simulink model "BEML_EMU"  (R2019b)
settings: configuration reference "ConfigSet_SimIntegration" (kept outside this file)
model workspace (MAT data in the model file):
  BrakesSampleTime = 0.01
  ConfigSampleTime = 0.05
  CouplingSampleTime = 0.05
  DoorsSampleTime = 0.05
  DynamicsSampleTime = 0.001
  ElectricalSampleTime = 0.05
  PRM_SimIntegration : Simulink.Parameter (value not decoded)
  PantographSampleTime = 0.05
  PneumaticsSampleTime = 0.01
  SampleTime = 0.001
  TractionSampleTime = 0.01
undefined symbols (not defined in the file): Acceleration, AngularAcceleration, AngularVelocity, BrakeFadeEnable, Brakes, BrakeShoeCoefficientCalculationMethod, BrakeShoeFrictionCoeff, BrakeTemperatureEnable, Common, DampingAdjustmentDesignMass, DavisCoeffA1, DavisCoeffA2, DavisCoeffB1, DavisCoeffB2, DavisCoefficients, DavisCoeffLeadCarC, DavisCoeffTailCarC, DiscIntNeverNeededParam, Doors, DragCalculationMethod, Dynamics, Effects, Electrical, EnableDampingAdjustmentByMass, Environment, Equipment, ExternalEffects, H, HasMotor, HasPanto, HornActivation, IsFirstVehicle, IsLastVehicle, isLeft, IsNonCab, LateralJolt, Location, LongitudinalJolt, MaxVehicles, MotionBaseSafetyCutout, OrientationDCM, P, Pantograph, Pneumatics, PneumaticsPoweredPanto, R, Traction, Transform, Tuning, UnitConfig, Velocity, VerticalJolt, VerticalJoltDown, VigilanceIntervention
libraries: simulink x35, IOStateMachinesLib x26, TestBenchLib x6, LatchesLib x3, BEML_EMU_BrakesInput_Lib x1, BEML_EMU_CBTCInterface_Lib x1, BEML_EMU_Couplers_Lib x1, BEML_EMU_DoorsInput_Lib x1, BEML_EMU_DynamicsInput_Lib x1, BEML_EMU_ElectricalInput_Lib x1, BEML_EMU_PantographInput_Lib x1, BEML_EMU_PneumaticsInput_Lib x1
(part 2 of 6)

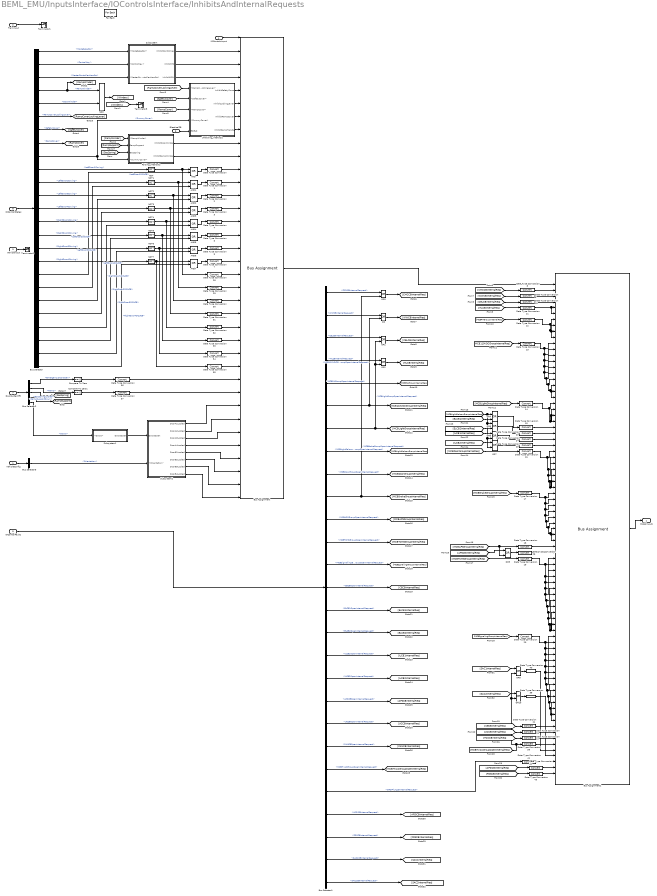
== system BEML_EMU/InputsInterface/IOControlsInterface/InhibitsAndInternalRequests ==
  VehicleConfig : Inport  Partition=on  PartitionDimension=1  PartitionWidth=1  PartitionOffset=0
  TrainInput : Inport  Port=2
  VehicleInput : Inport  Port=3  Partition=on  PartitionDimension=1  PartitionWidth=1  PartitionOffset=0
  IOControlsInput : Inport  Port=4  Partition=on  PartitionDimension=1  PartitionWidth=1  PartitionOffset=0
  IOControlFaults : Inport  Port=5  Partition=on  PartitionDimension=1  PartitionWidth=1  PartitionOffset=0
  ElectricalFB : Inport  Port=6  Partition=on  PartitionDimension=1  PartitionWidth=1  PartitionOffset=0
  DoorSystemFB : Inport  Port=7  Partition=on  PartitionDimension=1  PartitionWidth=1  PartitionOffset=0
  IOControlStates : Inport  Port=8  Partition=on  PartitionDimension=1  PartitionWidth=1  PartitionOffset=0
  AND{,1..7} (8 alike) : Logic  Operator=OR  AllPortsSameDT=off  OutDataTypeStr=boolean
  Bus Assignment : BusAssignment  AssignedSignals=ControlKey.Inhibit,ModeSelector.Inhibit,MasterControllerHandle.Inhibit,SafetyCover.Inhibit,RampCoverLockingLever.Inhibit,RampCover.Inhibit,RampHandle.Inhibit,DoorWinder.Inhibit,RampWinder.Inhibit,LeftDoor1EED.Inhibit,LeftDoor2EED.Inhibit,LeftDoor3EED.Inhibit,LeftDoor4EED.Inhibit,RightDoor1EED.Inhibit,RightDoor2EED.Inhibit,RightDoor3EED.Inhibit,RightDoor4EED.Inhibit,LeftDoor1DCUCB.Inhibit,LeftDoor2DCUCB.Inhibit,LeftDoor3DCUCB.Inhibit,LeftDoor4DCUCB.Inhibit,RightDoor1DCUCB.Inhibit,RightDoor2DCUCB.Inhibit,RightDoor3DCUCB.Inhibit,RightDoor4DCUCB.Inhibit,EmergencyDoorGasSpring.Inhibit,RampMiddleSupport.Inhibit,LeftDoor1Lockout.Inhibit,LeftDoor2Lockout.Inhibit,LeftDoor3Lockout.Inhibit,LeftDoor4Lockout.Inhibit,RightDoor1Lockout.Inhibit,RightDoor2Lockout.Inhibit,RightDoor3Lockout.Inhibit,RightDoor4Lockout.Inhibit
  Bus Assignment1 : BusAssignment  AssignedSignals=CMCCB.InternalRequest,WWCB.InternalRequest,CELCB.InternalRequest,HLLCB.InternalRequest,HLRCB.InternalRequest,OCCB1.InternalRequest,OCCB2.InternalRequest,PISCB1.InternalRequest,PISCB2.InternalRequest,TBCCB1.InternalRequest,TBCCB2.InternalRequest,SSICB.InternalRequest,HCB.InternalRequest,POCB.InternalRequest,TVDUCB.InternalRequest,ODDCB.InternalRequest,WIFICB.InternalRequest,WFLCB.InternalRequest,VCBCB.InternalRequest,MLCB.InternalRequest,TLLCB.InternalRequest,TLRCB.InternalRequest,CILCB.InternalRequest,ELCB1.InternalRequest,ELCB2.InternalRequest,ILCB1.InternalRequest,ILCB2.InternalRequest,LDRCB.InternalRequest,LDLCB.InternalRequest,DLCB.InternalRequest,DRCB.InternalRequest,LDICB.InternalRequest,DPLCB.InternalRequest,EDCB.InternalRequest,BLCB.InternalRequest,ZVBACB.InternalRequest,EBLR1CB.InternalRequest,EBLR2CB.InternalRequest,EBMVCB.InternalRequest,PBCB.InternalRequest,BECUCB1.InternalRequest,BECUCB2.InternalRequest,BECUCB3.InternalRequest,BCGCB.InternalRequest,APSCB.InternalRequest,TDICB.InternalRequest,ERCB.InternalRequest,TBNCB.InternalRequest,CSCCB.InternalRequest,CSBCB.InternalRequest,CSACB.InternalRequest,CDUCB.InternalRequest,DIOCB2.InternalRequest,DIOCB1.InternalRequest,SIOCB1.InternalRequest,SIOCB2.InternalRequest,RIO1CB.InternalRequest,RIO2CB.InternalRequest,TRIVCB.InternalRequest,VIO2CB.InternalRequest,VIO1CB.InternalRequest,PPU3CB.InternalRequest,PPU2CB.InternalRequest,PPU1CB.InternalRequest,C1CB.InternalRequest,NBCB.InternalRequest,MMCB.InternalRequest,CRSBCB.InternalRequest,DMICB.InternalRequest,TWVCB.InternalRequest,CBTCCB1.InternalRequest,NVICB.InternalRequest,CCNVIO1CB.InternalRequest,CECB.InternalRequest,VCCBOrUCCB.InternalRequest,PANCB.InternalRequest,CBFCCB.InternalRequest,SAC1CCB.InternalRequest,SAC2CCB.InternalRequest,ORDPlunger.InternalRequest,APSICB.InternalRequest,FDSCB.InternalRequest
  Bus Selector : BusSelector  OutputSignals=ModeSelector,ControlKey,MasterControllerHandle,RampWinder,DoorWinder,RampCoverLockingLever,SafetyCover,RampCover,DummyCover,LeftDoor1Coving,LeftDoor2Coving,LeftDoor3Coving,LeftDoor4Coving,RightDoor1Coving,RightDoor2Coving,RightDoor3Coving,RightDoor4Coving,LeftDoor1DCUCB,LeftDoor2DCUCB,LeftDoor3DCUCB,LeftDoor4DCUCB,RightDoor1DCUCB,RightDoor2DCUCB,RightDoor3DCUCB,RightDoor4DCUCB
  Bus Selector1 : BusSelector  OutputSignals=CCMCBInternalRequest,WWCBInternalRequest,CELCBInternalRequest,HLCBInternalRequest,MCBPAGroupOpenInternalRequest,MCB110VDCGroupOpenInternalRequest,MCBLightGroupOpenInternalRequest,MCBLightSaloonGroupOpenInternalRequest,MCBDoorGroupOpenInternalRequest,MCBBrakeGroupOpenInternalRequest,MCBAPSGroupOpenInternalRequest,MCBTCMSGroupOpenInternalRequest,MCBSignallingGroupOpenInternalRequest,CECBOpenInternalRequest,ELCB1OpenInternalRequest,ELCB2OpenInternalRequest,ILCB1OpenInternalRequest,ILCB2OpenInternalRequest,APSCBOpenInternalRequest,UCCBOpenInternalRequest,PANCBOpenInternalRequest,MCBHVACGroupOpenInternalRequest,ORDPlungerInternalRequest,APSICBInternalRequest,FDSCBInternalRequest,SAC1CBInternalRequest,SAC2CBInternalRequest
  Bus Selector2 : BusSelector  OutputSignals=EmergencyDoor.EmergencyDoorOpen,EmergencyDoor.Ramp,EmergencyDoor.GasSpringLocked,EmergencyDoor.RampSupportDown,Doors
  Bus Selector3 : BusSelector  OutputSignals=Common.Orientation
  Compare To Zero : simulink/Logic and Bit Operations/Compare To Zero  relop===  OutDataTypeStr=boolean
  Compare To Zero1 : simulink/Logic and Bit Operations/Compare To Zero  relop===  OutDataTypeStr=boolean
  Data Type Conversion{,1..43} (44 alike) : DataTypeConversion
  Folding_Interlocks : Subsystem
  For Each : ForEach  DisableCoverage=on
  NOR : Logic  Operator=NOR  AllPortsSameDT=off  OutDataTypeStr=boolean
  NOT{,1..7} (8 alike) : Logic  Operator=NOT  AllPortsSameDT=off  OutDataTypeStr=boolean
  OR{,1..10} (11 alike) : Logic  Operator=OR  AllPortsSameDT=off  OutDataTypeStr=boolean
  Subsystem : Subsystem
  Subsystem1 : Subsystem
  Subsystem2 : Subsystem
  Terminator1 : Terminator
  Terminator2 : Terminator
  Terminator3 : Terminator
  Unfolding_interlocks : Subsystem
  ModelInputs : Outport  ConcatenationDimension=1
  wires:
  AND4/1 -> Data Type Conversion4/1
  AND/1 -> Data Type Conversion/1
  IOControlStates/1 -> Bus Selector/1
  Bus Selector/17 -> NOT7/1  "<RightDoor4Coving>"
  Bus Selector/11 -> NOT1/1  "<LeftDoor2Coving>"
  AND5/1 -> Data Type Conversion5/1
  AND1/1 -> Data Type Conversion1/1
  AND6/1 -> Data Type Conversion6/1
  AND2/1 -> Data Type Conversion2/1
  AND3/1 -> Data Type Conversion3/1
  Bus Selector/10 -> NOT/1  "<LeftDoor1Coving>"
  Bus Selector/4 -> [RampWinder], NOR/1  "<RampWinder>"
  Bus Selector/13 -> NOT3/1  "<LeftDoor4Coving>"
  Bus Selector/12 -> NOT2/1  "<LeftDoor3Coving>"
  Bus Selector/14 -> NOT4/1  "<RightDoor1Coving>"
  Bus Selector/16 -> NOT6/1  "<RightDoor3Coving>"
  Bus Selector/15 -> NOT5/1  "<RightDoor2Coving>"
  AND7/1 -> Data Type Conversion7/1
  Folding_Interlocks/2(InhibitRampWinder) -> Bus Assignment/10
  Folding_Interlocks/1(InhibitDoorWinder) -> Bus Assignment/9
  Bus Assignment/1 -> Bus Assignment1/1
  IOControlFaults/1 -> Bus Selector1/1
  Subsystem/2(InhibitMS) -> Bus Assignment/3
  TrainInput/1 -> Terminator1/1
  Unfolding_interlocks/3(InhibitRampCover) -> Bus Assignment/7
  Bus Selector/2 -> Subsystem/2(<ControlKey>)  "<ControlKey>"
  Subsystem/1(InhibitControlKey) -> Bus Assignment/2
  VehicleInput/1 -> Terminator2/1
  VehicleConfig/1 -> Bus Selector3/1
  Bus Selector/5 -> NOR/2  "<DoorWinder>"
  Subsystem/3(InhibitMCH) -> Bus Assignment/4
  IOControlsInput/1 -> Bus Assignment/1
  Bus Selector/3 -> Subsystem/3(<MasterControllerHandle>)  "<MasterControllerHandle>"
  Unfolding_interlocks/1(InhibitSafetyCover) -> Bus Assignment/5
  Unfolding_interlocks/4(InhibitRampHandle) -> Bus Assignment/8
  Unfolding_interlocks/2(InhibitLockingLever) -> Bus Assignment/6
  Bus Selector/9 -> Unfolding_interlocks/4(<DummyCover>), Folding_Interlocks/4(<DummyCover>)  "<DummyCover>"
  Bus Selector/1 -> Subsystem/1(<ModeSelector>)  "<ModeSelector>"
  NOR/1 -> [Winders]
  [Winders] -> Terminator3/1
  [RampWinder] -> Folding_Interlocks/1(<RampWinder>)
  Bus Selector/6 -> [RampCoverLockingLever]  "<RampCoverLockingLever>"
  [RampCoverLockingLever] -> Unfolding_interlocks/1(<RampCoverLockingLever>)
  Bus Selector/7 -> [SafetyCover]  "<SafetyCover>"
  Bus Selector/8 -> [RampCover]  "<RampCover>"
  [SafetyCover] -> Unfolding_interlocks/2(<SafetyCover>)
  [RampCover] -> Unfolding_interlocks/3(<RampCover>)
  Data Type Conversion/1 -> Bus Assignment/11
  Data Type Conversion1/1 -> Bus Assignment/12
  Data Type Conversion2/1 -> Bus Assignment/13
  Data Type Conversion3/1 -> Bus Assignment/14
  Data Type Conversion4/1 -> Bus Assignment/15
  Data Type Conversion5/1 -> Bus Assignment/16
  Data Type Conversion6/1 -> Bus Assignment/17
  Data Type Conversion7/1 -> Bus Assignment/18
  Bus Selector1/1 -> OR3/1  "<CCMCBInternalRequest>"
  Data Type Conversion8/1 -> Bus Assignment1/2
  ElectricalFB/1 -> Unfolding_interlocks/5(EDELR)
  Bus Selector1/2 -> OR/1  "<WWCBInternalRequest>"
  Bus Selector1/3 -> OR1/1  "<CELCBInternalRequest>"
  Data Type Conversion9/1 -> Bus Assignment1/3
  Data Type Conversion10/1 -> Bus Assignment1/4
  Bus Selector1/4 -> OR2/1  "<HLCBInternalRequest>"
  Data Type Conversion11/1 -> Bus Assignment1/6, Bus Assignment1/5
  Bus Selector1/5 -> [MCBPAGroupInternalReq]  "<MCBPAGroupOpenInternalRequest>"
  Bus Assignment1/1 -> ModelInputs/1
  Bus Selector1/6 -> OR/2, [MCB110VDCGroupInternalReq]  "<MCB110VDCGroupOpenInternalRequest>"
  Bus Selector1/7 -> OR1/2, OR2/2, [MCBLightGroupInternalReq]  "<MCBLightGroupOpenInternalRequest>"
  Bus Selector1/8 -> [MCBLightSaloonGroupInternalReq]  "<MCBLightSaloonGroupOpenInternalRequest>"
  Bus Selector1/9 -> [MCBDoorGroupInternalReq]  "<MCBDoorGroupOpenInternalRequest>"
  Bus Selector1/10 -> OR3/2, [MCBBrakeGroupInternalReq]  "<MCBBrakeGroupOpenInternalRequest>"
  Bus Selector1/11 -> [MCBAPSGroupInternalReq]  "<MCBAPSGroupOpenInternalRequest>"
  Bus Selector1/12 -> [MCBTCMSGroupInternalReq]  "<MCBTCMSGroupOpenInternalRequest>"
  Bus Selector1/13 -> [MCBSgnalingGroupInternalReq]  "<MCBSignallingGroupOpenInternalRequest>"
  OR/1 -> [WWCBInternalReq]
  OR1/1 -> [CELCBInternalReq]
  OR2/1 -> [HLCBInternalReq]
  OR3/1 -> [CMCCBInternalReq]
  [CMCCBInternalReq] -> Data Type Conversion8/1
  [WWCBInternalReq] -> Data Type Conversion9/1
  [HLCBInternalReq] -> Data Type Conversion11/1
  [CELCBInternalReq] -> Data Type Conversion10/1
  [MCBPAGroupInternalReq] -> Data Type Conversion12/1
  Data Type Conversion12/1 -> Bus Assignment1/9, Bus Assignment1/10, Bus Assignment1/8, Bus Assignment1/7
  [MCB110VDCGroupInternalReq] -> Data Type Conversion13/1
  Data Type Conversion13/1 -> Bus Assignment1/18, Bus Assignment1/19, Bus Assignment1/20, Bus Assignment1/17, Bus Assignment1/16, Bus Assignment1/15, Bus Assignment1/14, Bus Assignment1/13, Bus Assignment1/12, Bus Assignment1/11
  [MCBLightGroupInternalReq] -> Data Type Conversion14/1
  Data Type Conversion14/1 -> Bus Assignment1/22, Bus Assignment1/23, Bus Assignment1/24, Bus Assignment1/21
  OR4/1 -> Data Type Conversion15/1
  [MCBDoorGroupInternalReq] -> Data Type Conversion16/1
  Data Type Conversion16/1 -> Bus Assignment1/30, Bus Assignment1/31, Bus Assignment1/32, Bus Assignment1/33, Bus Assignment1/35, Bus Assignment1/34, Bus Assignment1/29
  [MCBBrakeGroupInternalReq] -> Data Type Conversion17/1
  Data Type Conversion17/1 -> Bus Assignment1/38, Bus Assignment1/40, Bus Assignment1/41, Bus Assignment1/42, Bus Assignment1/43, Bus Assignment1/44, Bus Assignment1/39, Bus Assignment1/37, Bus Assignment1/36
  [MCBAPSGroupInternalReq] -> OR9/2, Data Type Conversion18/1
  Data Type Conversion18/1 -> Bus Assignment1/45
  [MCBTCMSGroupInternalReq] -> Data Type Conversion19/1
  Data Type Conversion19/1 -> Bus Assignment1/48, Bus Assignment1/49, Bus Assignment1/50, Bus Assignment1/51, Bus Assignment1/52, Bus Assignment1/53, Bus Assignment1/54, Bus Assignment1/55, Bus Assignment1/56, Bus Assignment1/57, Bus Assignment1/58, Bus Assignment1/59, Bus Assignment1/47
  Data Type Conversion20/1 -> Bus Assignment1/62, Bus Assignment1/63, Bus Assignment1/64, Bus Assignment1/65, Bus Assignment1/66, Bus Assignment1/67, Bus Assignment1/68, Bus Assignment1/69, Bus Assignment1/70, Bus Assignment1/71, Bus Assignment1/73, Bus Assignment1/72, Bus Assignment1/74, Bus Assignment1/61, Bus Assignment1/60
  [MCBSgnalingGroupInternalReq] -> Data Type Conversion20/1
  Bus Selector1/14 -> [CECBInternalReq]  "<CECBOpenInternalRequest>"
  Bus Selector1/15 -> [ELCB1InternalReq]  "<ELCB1OpenInternalRequest>"
  Bus Selector1/16 -> [ELCB2InternalReq]  "<ELCB2OpenInternalRequest>"
  Bus Selector1/17 -> [ILCB1InternalReq]  "<ILCB1OpenInternalRequest>"
  Bus Selector1/18 -> [ILCB2InternalReq]  "<ILCB2OpenInternalRequest>"
  Bus Selector1/19 -> [APSCBInternalReq]  "<APSCBOpenInternalRequest>"
  Bus Selector1/20 -> [UCCBInternalReq]  "<UCCBOpenInternalRequest>"
  [CECBInternalReq] -> Data Type Conversion21/1
  Data Type Conversion21/1 -> Bus Assignment1/75
  [UCCBInternalReq] -> Data Type Conversion22/1
  Data Type Conversion22/1 -> Bus Assignment1/76
  Data Type Conversion15/1 -> Bus Assignment1/25
  Data Type Conversion23/1 -> Bus Assignment1/26
  Data Type Conversion24/1 -> Bus Assignment1/27
  Data Type Conversion25/1 -> Bus Assignment1/28
  OR5/1 -> Data Type Conversion23/1
  OR6/1 -> Data Type Conversion24/1
  OR7/1 -> Data Type Conversion25/1
  [MCBLightSaloonGroupInternalReq] -> OR7/2, OR6/2, OR5/1, OR4/1
  [ELCB1InternalReq] -> OR4/2
  [ELCB2InternalReq] -> OR5/2
  [ILCB1InternalReq] -> OR6/1
  [ILCB2InternalReq] -> OR7/1
  Data Type Conversion26/1 -> Bus Assignment1/46
  OR9/1 -> Data Type Conversion26/1
  [APSCBInternalReq] -> OR9/1
  Bus Selector1/21 -> [PANCBInternalReq]  "<PANCBOpenInternalRequest>"
  [PANCBInternalReq] -> Data Type Conversion27/1
  Data Type Conversion27/1 -> Bus Assignment1/77
  Bus Selector/18 -> AND/2  "<LeftDoor1DCUCB>"
  Bus Selector/19 -> AND1/2  "<LeftDoor2DCUCB>"
  Bus Selector/20 -> AND2/2  "<LeftDoor3DCUCB>"
  Bus Selector/21 -> AND3/2  "<LeftDoor4DCUCB>"
  Bus Selector/22 -> AND4/2  "<RightDoor1DCUCB>"
  Bus Selector/23 -> AND5/2  "<RightDoor2DCUCB>"
  Bus Selector/24 -> AND6/2  "<RightDoor3DCUCB>"
  Bus Selector/25 -> AND7/2  "<RightDoor4DCUCB>"
  NOT/1 -> Data Type Conversion28/1, AND/1
  NOT1/1 -> Data Type Conversion29/1, AND1/1
  NOT2/1 -> Data Type Conversion30/1, AND2/1
  NOT3/1 -> Data Type Conversion31/1, AND3/1
  NOT4/1 -> Data Type Conversion32/1, AND4/1
  NOT5/1 -> Data Type Conversion33/1, AND5/1
  NOT6/1 -> Data Type Conversion34/1, AND6/1
  NOT7/1 -> Data Type Conversion35/1, AND7/1
  Data Type Conversion28/1 -> Bus Assignment/19
  Data Type Conversion29/1 -> Bus Assignment/20
  Data Type Conversion30/1 -> Bus Assignment/21
  Data Type Conversion31/1 -> Bus Assignment/22
  Data Type Conversion32/1 -> Bus Assignment/23
  Data Type Conversion33/1 -> Bus Assignment/24
  Data Type Conversion34/1 -> Bus Assignment/25
  Data Type Conversion35/1 -> Bus Assignment/26
  [RampSupport] -> Folding_Interlocks/2(RampSupport)
  [GasSpring] -> Folding_Interlocks/3(GasSpring)
  Compare To Zero/1 -> Data Type Conversion36/1
  Compare To Zero1/1 -> Data Type Conversion37/1
  Data Type Conversion36/1 -> Bus Assignment/27
  Data Type Conversion37/1 -> Bus Assignment/28
  Bus Selector1/22 -> [MCBHVACGroupOpenInternalReq]  "<MCBHVACGroupOpenInternalRequest>"
  Data Type Conversion39/1 -> Bus Assignment1/78
  DoorSystemFB/1 -> Bus Selector2/1
  Bus Selector2/1 -> Compare To Zero/1  "<EmergencyDoorOpen>"
  Bus Selector2/2 -> Compare To Zero1/1  "<Ramp>"
  Bus Selector2/3 -> [GasSpring]  "<GasSpringLocked>"
  Bus Selector2/4 -> [RampSupport]  "<RampSupportDown>"
  Bus Selector2/5 -> Subsystem1/1(<Doors>)  "<Doors>"
  Subsystem1/1(DoorsOpen) -> Subsystem2/1(DoorsOpen)
  Bus Selector3/1 -> Subsystem2/2(<Orientation>)  "<Orientation>"
  Subsystem2/1(DoorA1Locked) -> Bus Assignment/29
  Subsystem2/2(DoorA2Locked) -> Bus Assignment/30
  Subsystem2/3(DoorA3Locked) -> Bus Assignment/31
  Subsystem2/4(DoorA4Locked) -> Bus Assignment/32
  Subsystem2/5(DoorB1Locked) -> Bus Assignment/33
  Subsystem2/6(DoorB2Locked) -> Bus Assignment/34
  Subsystem2/7(DoorB3Locked) -> Bus Assignment/35
  Subsystem2/8(DoorB4Locked) -> Bus Assignment/36
  Bus Selector1/23 -> Data Type Conversion41/1  "<ORDPlungerInternalRequest>"
  Data Type Conversion41/1 -> Bus Assignment1/81
  Bus Selector1/24 -> [APSICBInternalReq]  "<APSICBInternalRequest>"
  Bus Selector1/25 -> [FDSCBInternalReq]  "<FDSCBInternalRequest>"
  Bus Selector1/26 -> [SAC1InternalReq]  "<SAC1CBInternalRequest>"
  Bus Selector1/27 -> [SAC2InternalReq]  "<SAC2CBInternalRequest>"
  [APSICBInternalReq] -> Data Type Conversion42/1
  [FDSCBInternalReq] -> Data Type Conversion43/1
  [SAC1InternalReq] -> OR8/1
  [SAC2InternalReq] -> OR10/1
  OR8/1 -> Data Type Conversion40/1
  OR10/1 -> Data Type Conversion38/1
  [MCBHVACGroupOpenInternalReq] -> OR10/2, OR8/2, Data Type Conversion39/1
  Data Type Conversion38/1 -> Bus Assignment1/80
  Data Type Conversion40/1 -> Bus Assignment1/79
  Data Type Conversion42/1 -> Bus Assignment1/82
  Data Type Conversion43/1 -> Bus Assignment1/83

== system BEML_EMU/InputsInterface/VehicleConfigProcessing/VehicleConfigInterface ==
  VehicleConfig : Inport
  TrainInput : Inport  Port=2
  Enable : EnablePort
  Data Type Conversion : DataTypeConversion
  Enumerated Voltages : VectorOperationsLib/Enumerated Voltages
      settings: SourceProductName=Sydac Utilities
  Max : MinMax  Function=max
  Product : Product
  Terminator : Terminator
  Unit Delay : UnitDelay  SampleTime=-1  HasFrameUpgradeWarning=on
  VehicleConfigInterface : Subsystem
  VehicleEnabled : Subsystem
  VehicleConfigProcessed : Outport  SourceOfInitialOutputValue=Input signal  VectorParamsAs1DForOutWhenUnconnected=off
  wires:
  VehicleConfigInterface/1(VehicleConfigProcessed) -> VehicleConfigProcessed/1
  VehicleConfig/1 -> VehicleEnabled/1(VehicleConfig), VehicleConfigInterface/1(VehicleConfig)
  TrainInput/1 -> VehicleConfigInterface/6(TrainInput)
  VehicleEnabled/2(VehicleEnabledDown) -> VehicleConfigInterface/3(VehicleDownEnabled)
  VehicleEnabled/1(VehicleEnabledUp) -> VehicleConfigInterface/2(VehicleUpEnabled)
  VehicleConfigInterface/3(UnitConn) -> Enumerated Voltages/1
  Enumerated Voltages/1 -> Product/2
  Product/1 -> Data Type Conversion/1
  VehicleEnabled/3(VehicleClassDown) -> VehicleConfigInterface/4(ClassDown)
  VehicleEnabled/4(VehicleClassUp) -> VehicleConfigInterface/5(ClassUp)
  Unit Delay/1 -> VehicleConfigInterface/7(UnitID), Max/1
  VehicleConfigInterface/2(Enable) -> Product/1
  Data Type Conversion/1 -> Terminator/1, Unit Delay/1
  Max/1 -> VehicleConfigInterface/8(MaxUnits)

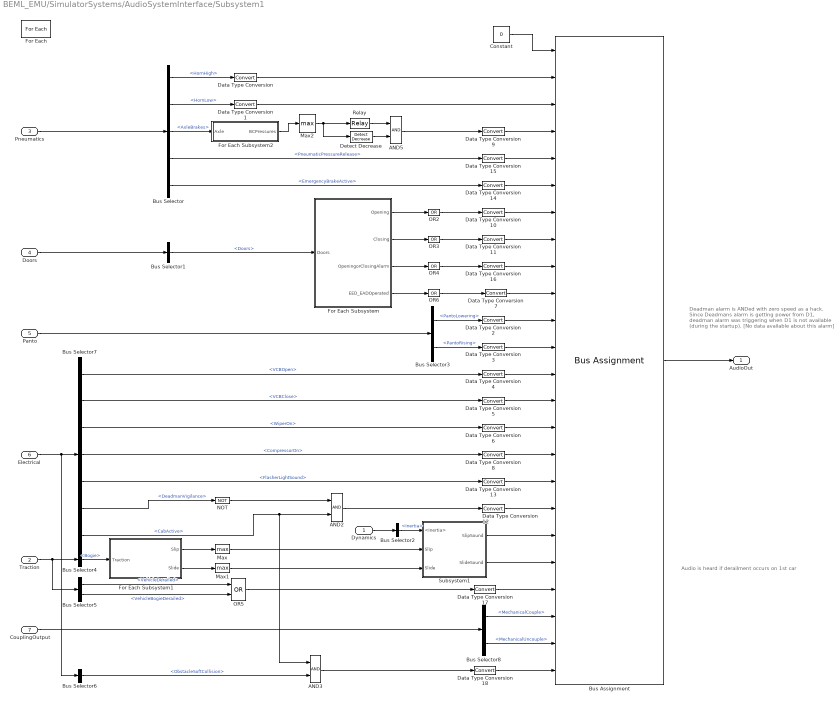
== system BEML_EMU/SimulatorSystems/AudioSystemInterface/Subsystem1 ==
  note: Audio is heard if derailment occurs on 1st car
  note: Deadman alarm is ANDed with zero speed as a hack.
      | Since Deadmans alarm is getting power from D1,
      | deadman alarm was triggering when D1
      | is not available (during the startup).
      | [No data available about this alarm]
  Dynamics : Inport  Partition=on  PartitionDimension=1  PartitionWidth=1  PartitionOffset=0
  Traction : Inport  Port=2  Partition=on  PartitionDimension=1  PartitionWidth=1  PartitionOffset=0
  Pneumatics : Inport  Port=3  Partition=on  PartitionDimension=1  PartitionWidth=1  PartitionOffset=0
  Doors : Inport  Port=4  Partition=on  PartitionDimension=1  PartitionWidth=1  PartitionOffset=0
  Panto : Inport  Port=5  Partition=on  PartitionDimension=1  PartitionWidth=1  PartitionOffset=0
  Electrical : Inport  Port=6  Partition=on  PartitionDimension=1  PartitionWidth=1  PartitionOffset=0
  CouplingOutput : Inport  Port=7  Partition=on  PartitionDimension=1  PartitionWidth=1  PartitionOffset=0
  AND2 : Logic  AllPortsSameDT=off  OutDataTypeStr=boolean
  AND3 : Logic  AllPortsSameDT=off  OutDataTypeStr=boolean
  AND5 : Logic  AllPortsSameDT=off  OutDataTypeStr=boolean
  Bus Assignment : BusAssignment  AssignedSignals=HornHigh,HornLow,AirBrakeRelease,PneumaticPressureRelease,EmergencyBrakeApplicationSound,SaloonDoorOpeningBuzzer,SaloonDoorClosingBuzzer,DoorWarningBuzzer,EEDEADOperated,PantographLowering,PantographRaising,VCBOpenSound,VCBCloseSound,WiperSound,CompressorStartAndRunSound,FlasherLightOperationSound,DeadmanAlarm,WheelSlip,WheelSlide,Derailment,CollisionDetectionCoupling,MechanicalUncouple,ObstacleSoftCollision
  Bus Selector : BusSelector  OutputSignals=Audio.HornHigh,Audio.HornLow,AxleBrakes,Audio.PneumaticPressureRelease,Audio.EmergencyBrakeActive
  Bus Selector1 : BusSelector  OutputSignals=Doors
  Bus Selector2 : BusSelector  OutputSignals=Inertia
  Bus Selector3 : BusSelector  OutputSignals=PantoLowering,PantoRising
  Bus Selector4 : BusSelector  OutputSignals=TractionControl.TCMS.Bogie
  Bus Selector5 : BusSelector  OutputSignals=TractionControl.TCMS.VehicleDerailed,TractionControl.TCMS.VehicleBogieDerailed
  Bus Selector6 : BusSelector  OutputSignals=Audio.ObstacleSoftCollision
  Bus Selector7 : BusSelector  OutputSignals=Audio.VCBOpen,Audio.VCBClose,Audio.WiperOn,Audio.CompressorOn,Audio.FlasherLightSound,Audio.DeadmanVigilance,TCMS.CabActive
  Bus Selector8 : BusSelector  OutputSignals=CouplerAudio.MechanicalCouple,CouplerAudio.MechanicalUncouple
  Constant : Constant  Value=0  OutDataTypeStr=Bus: BD_SimIntegration_Out_Vehicle_Audio
  Data Type Conversion{,1..18} (19 alike) : DataTypeConversion
  Detect Decrease : simulink/Logic and Bit Operations/Detect Decrease  vinit=0.0  OutDataTypeStr=boolean
  For Each : ForEach  DisableCoverage=on
  For Each Subsystem : Subsystem  TreatAsAtomicUnit=on
  For Each Subsystem1 : Subsystem  TreatAsAtomicUnit=on
  For Each Subsystem2 : Subsystem  TreatAsAtomicUnit=on
  Max : MinMax  Function=max
  Max1 : MinMax  Function=max
  Max2 : MinMax  Function=max
  NOT : Logic  Operator=NOT  AllPortsSameDT=off  OutDataTypeStr=boolean
  OR{2..4,6} (4 alike) : Logic  Operator=OR  Inputs=1  AllPortsSameDT=off  OutDataTypeStr=boolean
  OR5 : Logic  Operator=OR  AllPortsSameDT=off  OutDataTypeStr=boolean
  Relay : Relay  OnSwitchValue=3.0e5  OffSwitchValue=2.0e5
  Subsystem1 : Subsystem
  AudioOut : Outport  ConcatenationDimension=1
  wires:
  Bus Selector7/5 -> Data Type Conversion13/1  "<FlasherLightSound>"
  CouplingOutput/1 -> Bus Selector8/1
  AND2/1 -> Data Type Conversion12/1
  Dynamics/1 -> Bus Selector2/1
  Data Type Conversion16/1 -> Bus Assignment/9
  Data Type Conversion10/1 -> Bus Assignment/7
  OR4/1 -> Data Type Conversion16/1
  Electrical/1 -> Bus Selector6/1, Bus Selector7/1
  Bus Selector7/1 -> Data Type Conversion4/1  "<VCBOpen>"
  Data Type Conversion11/1 -> Bus Assignment/8
  For Each Subsystem/2(Closing) -> OR3/1
  For Each Subsystem/3(OpeningorClosingAlarm) -> OR4/1
  Data Type Conversion14/1 -> Bus Assignment/6
  Bus Selector/4 -> Data Type Conversion15/1  "<PneumaticPressureRelease>"
  Bus Selector7/3 -> Data Type Conversion6/1  "<WiperOn>"
  NOT/1 -> AND2/1
  Bus Selector7/6 -> NOT/1  "<DeadmanVigilance>"
  Bus Selector3/1 -> Data Type Conversion2/1  "<PantoLowering>"
  Bus Selector7/2 -> Data Type Conversion5/1  "<VCBClose>"
  OR3/1 -> Data Type Conversion11/1
  Traction/1 -> Bus Selector5/1, Bus Selector4/1
  OR2/1 -> Data Type Conversion10/1
  Bus Selector/5 -> Data Type Conversion14/1  "<EmergencyBrakeActive>"
  AND5/1 -> Data Type Conversion9/1
  Bus Selector/3 -> For Each Subsystem2/1(Axle)  "<AxleBrakes>"
  For Each Subsystem2/1(BCPressures) -> Max2/1
  Panto/1 -> Bus Selector3/1
  For Each Subsystem/1(Opening) -> OR2/1
  For Each Subsystem1/2(Slide) -> Max1/1
  Bus Selector3/2 -> Data Type Conversion3/1  "<PantoRising>"
  Bus Selector1/1 -> For Each Subsystem/1(Doors)  "<Doors>"
  Doors/1 -> Bus Selector1/1
  For Each Subsystem1/1(Slip) -> Max/1
  Bus Selector7/4 -> Data Type Conversion8/1  "<CompressorOn>"
  Data Type Conversion1/1 -> Bus Assignment/3
  Constant/1 -> Bus Assignment/1
  Data Type Conversion/1 -> Bus Assignment/2
  Bus Assignment/1 -> AudioOut/1
  Bus Selector/1 -> Data Type Conversion/1  "<HornHigh>"
  Bus Selector/2 -> Data Type Conversion1/1  "<HornLow>"
  Bus Selector7/7 -> AND3/1, AND2/2  "<CabActive>"
  Bus Selector5/1 -> OR5/1  "<VehicleDerailed>"
  Bus Selector5/2 -> OR5/2  "<VehicleBogieDerailed>"
  OR5/1 -> Data Type Conversion17/1
  Bus Selector4/1 -> For Each Subsystem1/1(Traction)  "<Bogie>"
  Bus Selector2/1 -> Subsystem1/1(<Inertia>)  "<Inertia>"
  Max/1 -> Subsystem1/2(Slip)
  Max1/1 -> Subsystem1/3(Slide)
  For Each Subsystem/4(EED_EADOperated) -> OR6/1
  Data Type Conversion7/1 -> Bus Assignment/10
  OR6/1 -> Data Type Conversion7/1
  Data Type Conversion2/1 -> Bus Assignment/11
  Data Type Conversion3/1 -> Bus Assignment/12
  Data Type Conversion4/1 -> Bus Assignment/13
  Data Type Conversion5/1 -> Bus Assignment/14
  Data Type Conversion6/1 -> Bus Assignment/15
  Data Type Conversion8/1 -> Bus Assignment/16
  Data Type Conversion13/1 -> Bus Assignment/17
  Data Type Conversion12/1 -> Bus Assignment/18
  Subsystem1/1(SlipSound) -> Bus Assignment/19
  Subsystem1/2(SlideSound) -> Bus Assignment/20
  Data Type Conversion17/1 -> Bus Assignment/21
  Bus Selector8/1 -> Bus Assignment/22  "<MechanicalCouple>"
  Bus Selector8/2 -> Bus Assignment/23  "<MechanicalUncouple>"
  Bus Selector6/1 -> AND3/2  "<ObstacleSoftCollision>"
  AND3/1 -> Data Type Conversion18/1
  Data Type Conversion18/1 -> Bus Assignment/24
  Pneumatics/1 -> Bus Selector/1
  Detect Decrease/1 -> AND5/2
  Relay/1 -> AND5/1
  Data Type Conversion15/1 -> Bus Assignment/5
  Max2/1 -> Detect Decrease/1, Relay/1
  Data Type Conversion9/1 -> Bus Assignment/4

== system BEML_EMU/SimulatorSystems/ScoringSystemInterface/TrainLevelScoring ==
  note: Total Energy Consumption = Total Traction Energy Consumed - Total ED Braking Energy Regenerated + Constant Base Load for powering Auxiliary Devices
  In Bus Element : Inport  PortName=TractionOut
  In Bus Element2 : Inport  Port=2  PortName=ElectricalVehicleOut
  Abs : Abs
  Abs1 : Abs
  Add : Sum  Inputs=+-+
  Bus Assignment : BusAssignment  AssignedSignals=TotalEnergyConsumption
  Constant : Constant  Value=5000
  Constant1 : Constant  Value=0  OutDataTypeStr=Bus: BD_SimIntegration_Out_Train_Scoring
  Constant2 : Constant  Value=0
  Discrete-Time Integrator : DiscreteIntegrator  SampleTime=-1  ICPrevOutput=DiscIntNeverNeededParam  ICPrevScaledInput=DiscIntNeverNeededParam
  For Each Subsystem : Subsystem  TreatAsAtomicUnit=on
  For Each Subsystem1 : Subsystem  TreatAsAtomicUnit=on
  Sum of Elements : Sum  Inputs=+
  Sum of Elements1 : Sum  Inputs=+
  Sum of Elements2 : Sum  Inputs=+
  Switch : Switch  Criteria=u2 > Threshold
  Out1 : Outport
  wires:
  Bus Assignment/1 -> Out1/1
  For Each Subsystem/1(VehicleTractiveEnergy) -> Abs/1
  Constant1/1 -> Bus Assignment/1
  In Bus Element/1 -> For Each Subsystem/1(In1)
  Sum of Elements/1 -> Add/1
  Abs/1 -> Sum of Elements/1
  Add/1 -> Bus Assignment/2
  Abs1/1 -> Sum of Elements1/1
  Sum of Elements1/1 -> Add/2
  For Each Subsystem/2(VehicleEDBrakingEnergy) -> Abs1/1
  For Each Subsystem1/1(Out1) -> Sum of Elements2/1
  Switch/1 -> Discrete-Time Integrator/1  "AuxPower"
  Constant/1 -> Switch/1
  Constant2/1 -> Switch/3
  Sum of Elements2/1 -> Switch/2
  Discrete-Time Integrator/1 -> Add/3  "AuxEnergyConsumed"
  In Bus Element2/1 -> For Each Subsystem1/1(In1)

== system BEML_EMU/SimulatorSystems/ScoringSystemInterface/VehicleLevelScoring ==
  ElectricalOut : Inport  Partition=on  PartitionDimension=1  PartitionWidth=1  PartitionOffset=0
  PneumaticsVehicleOut : Inport  Port=2  Partition=on  PartitionDimension=1  PartitionWidth=1  PartitionOffset=0
  Bus Assignment : BusAssignment  AssignedSignals=VigilanceIntervention,HornActivation
  Bus Selector : BusSelector  OutputSignals=TCMS.CabActive,SignalSys.ATOMode,SignalSys.ATBMode,SignalSys.UTOMode,Scoring.DeadmanRelay
  Bus Selector1 : BusSelector  OutputSignals=Audio.HornHigh,Audio.HornLow
  Constant1 : Constant  Value=0  OutDataTypeStr=Bus: BD_SimIntegration_Out_Vehicle_Scoring
  Data Type Conversion : DataTypeConversion
  Data Type Conversion1 : DataTypeConversion
  For Each : ForEach  DisableCoverage=on
  Logical Operator : Logic  Inputs=5  AllPortsSameDT=off  OutDataTypeStr=boolean
  Logical Operator{1..4} (4 alike) : Logic  Operator=NOT  AllPortsSameDT=off  OutDataTypeStr=boolean
  OR : Logic  Operator=OR  AllPortsSameDT=off  OutDataTypeStr=boolean
  Scoring : Outport  ConcatenationDimension=1
  wires:
  Bus Assignment/1 -> Scoring/1
  ElectricalOut/1 -> Bus Selector/1
  Constant1/1 -> Bus Assignment/1
  Bus Selector/1 -> Logical Operator/1  "<CabActive>"
  Logical Operator1/1 -> Logical Operator/2
  Bus Selector/2 -> Logical Operator1/1  "<ATOMode>"
  Logical Operator2/1 -> Logical Operator/3
  Bus Selector/3 -> Logical Operator2/1  "<ATBMode>"
  Logical Operator3/1 -> Logical Operator/4
  Bus Selector/4 -> Logical Operator3/1  "<UTOMode>"
  Logical Operator4/1 -> Logical Operator/5
  Bus Selector/5 -> Logical Operator4/1  "<DeadmanRelay>"
  Logical Operator/1 -> Data Type Conversion/1
  Data Type Conversion/1 -> Bus Assignment/2
  PneumaticsVehicleOut/1 -> Bus Selector1/1
  Bus Selector1/1 -> OR/1  "<HornHigh>"
  OR/1 -> Data Type Conversion1/1
  Bus Selector1/2 -> OR/2  "<HornLow>"
  Data Type Conversion1/1 -> Bus Assignment/3

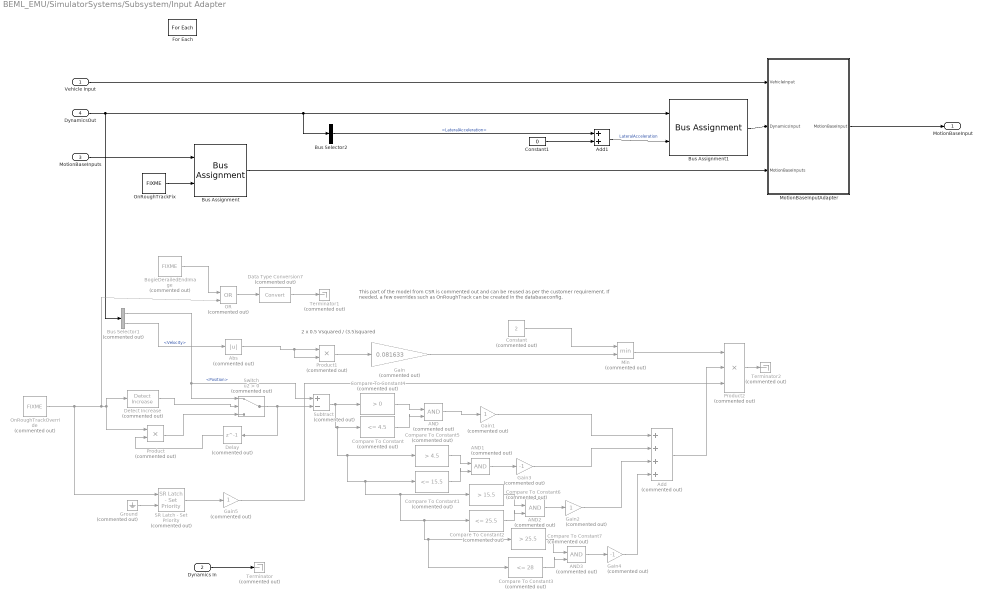
== system BEML_EMU/SimulatorSystems/Subsystem/Input Adapter ==
  note: This part of the model from CSR is commented out and can be reused as per the customer requirement.
      | If needed, a few overrides such as OnRoughTrack can be created in the databaseconfig.
  note: 2 x 0.5 Vsquared / (3.5)squared
  Vehicle Input : Inport  Partition=on  PartitionDimension=1  PartitionWidth=1  PartitionOffset=0
  Dynamics In : Inport  Port=2  Partition=on  PartitionDimension=1  PartitionWidth=1  PartitionOffset=0
  MotionBaseInputs : Inport  Port=3  Partition=on  PartitionDimension=1  PartitionWidth=1  PartitionOffset=0
  DynamicsOut : Inport  Port=4  Partition=on  PartitionDimension=1  PartitionWidth=1  PartitionOffset=0
  AND{,1..3} (4 alike) : Logic  Commented=on  IconShape=distinctive  AllPortsSameDT=off  OutDataTypeStr=boolean
  Abs : Abs  Commented=on
  Add : Sum  Commented=on  Inputs=4
  Add1 : Sum
  BogieDerailedEndImage : TestBenchLib/FIXME  Commented=on
      settings: SourceProductName=Sydac Utilities
  Bus Assignment : BusAssignment  AssignedSignals=Effects.OnRoughTrack
  Bus Assignment1 : BusAssignment  AssignedSignals=TrackGeometry.LateralAcceleration
  Bus Selector1 : BusSelector  Commented=on  OutputSignals=Inertia.Position,Inertia.Velocity
  Bus Selector2 : BusSelector  OutputSignals=TrackGeometry.LateralAcceleration
  Compare To Constant : simulink/Logic and Bit Operations/Compare To Constant  Commented=on  relop=<=  const=4.5  OutDataTypeStr=boolean
  Compare To Constant1 : simulink/Logic and Bit Operations/Compare To Constant  Commented=on  relop=<=  const=15.5  OutDataTypeStr=boolean
  Compare To Constant2 : simulink/Logic and Bit Operations/Compare To Constant  Commented=on  relop=<=  const=25.5  OutDataTypeStr=boolean
  Compare To Constant3 : simulink/Logic and Bit Operations/Compare To Constant  Commented=on  relop=<=  const=28  OutDataTypeStr=boolean
  Compare To Constant4 : simulink/Logic and Bit Operations/Compare To Constant  Commented=on  relop=>  const=0  OutDataTypeStr=boolean
  Compare To Constant5 : simulink/Logic and Bit Operations/Compare To Constant  Commented=on  relop=>  const=4.5  OutDataTypeStr=boolean
  Compare To Constant6 : simulink/Logic and Bit Operations/Compare To Constant  Commented=on  relop=>  const=15.5  OutDataTypeStr=boolean
  Compare To Constant7 : simulink/Logic and Bit Operations/Compare To Constant  Commented=on  relop=>  const=25.5  OutDataTypeStr=boolean
  Constant : Constant  Commented=on  Value=2
  Constant1 : Constant  Value=0
  Data Type Conversion7 : DataTypeConversion  Commented=on
  Delay : Delay  Commented=on  DelayLength=1
  Detect Increase : simulink/Logic and Bit Operations/Detect Increase  Commented=on  vinit=0.0  OutDataTypeStr=boolean
  For Each : ForEach  DisableCoverage=on
  Gain : Gain  Commented=on  Gain=0.081633
  Gain1 : Gain  Commented=on
  Gain2 : Gain  Commented=on
  Gain3 : Gain  Commented=on  Gain=-1
  Gain4 : Gain  Commented=on  Gain=-1
  Gain5 : Gain  Commented=on
  Ground : Ground  Commented=on
  Min : MinMax  Commented=on  Inputs=2
  MotionBaseInputAdapter : Subsystem
  OR : Logic  Commented=on  Operator=OR  IconShape=distinctive  AllPortsSameDT=off  OutDataTypeStr=boolean
  OnRoughTrackFix : TestBenchLib/FIXME
      settings: SourceProductName=Sydac Utilities
  OnRoughTrackOverride : TestBenchLib/FIXME  Commented=on
      settings: SourceProductName=Sydac Utilities
  Product : Product  Commented=on
  Product1 : Product  Commented=on
  Product2 : Product  Commented=on  Inputs=3
  SR Latch - Set Priority : LatchesLib/SR Latch - Set Priority  Commented=on  initial_condition=0
      settings: SourceProductName=Latches
  Subtract : Sum  Commented=on  Inputs=+-
  Switch : Switch  Commented=on  Criteria=u2 > Threshold
  Terminator : Terminator  Commented=on
  Terminator1 : Terminator  Commented=on
  Terminator2 : Terminator  Commented=on
  MotionBaseInput : Outport  ConcatenationDimension=1
  wires:
  MotionBaseInputAdapter/1(MotionBaseInput) -> MotionBaseInput/1
  DynamicsOut/1 -> Bus Selector1/1, Bus Selector2/1, Bus Assignment1/1
  Vehicle Input/1 -> MotionBaseInputAdapter/1(VehicleInput)
  MotionBaseInputs/1 -> Bus Assignment/1
  Bus Assignment/1 -> MotionBaseInputAdapter/3(MotionBaseInputs)
  Data Type Conversion7/1 -> Terminator1/1
  OnRoughTrackOverride/1 -> SR Latch - Set Priority/1, OR/2, Product/1, Detect Increase/1
  Bus Selector1/1 -> Switch/1, Subtract/1  "<Position>"
  Switch/1 -> Subtract/2, Delay/1
  Delay/1 -> Product/2
  Detect Increase/1 -> Switch/2
  Product/1 -> Switch/3
  Subtract/1 -> Compare To Constant3/1, Compare To Constant7/1, Compare To Constant2/1, Compare To Constant6/1, Compare To Constant1/1, Compare To Constant5/1, Compare To Constant/1, Compare To Constant4/1
  Compare To Constant4/1 -> AND/1
  Compare To Constant/1 -> AND/2
  Compare To Constant5/1 -> AND1/1
  Compare To Constant1/1 -> AND1/2
  Compare To Constant6/1 -> AND2/1
  Compare To Constant2/1 -> AND2/2
  Compare To Constant7/1 -> AND3/1
  Compare To Constant3/1 -> AND3/2
  Bus Selector1/2 -> Abs/1  "<Velocity>"
  Abs/1 -> Product1/2, Product1/1
  Product1/1 -> Gain/1
  AND/1 -> Gain1/1
  AND2/1 -> Gain2/1
  AND1/1 -> Gain3/1
  AND3/1 -> Gain4/1
  Gain1/1 -> Add/1
  Gain3/1 -> Add/2
  Gain2/1 -> Add/3
  Gain4/1 -> Add/4
  Gain/1 -> Min/2
  Add/1 -> Product2/2
  Bus Selector2/1 -> Add1/1  "<LateralAcceleration>"
  Product2/1 -> Terminator2/1
  Add1/1 -> Bus Assignment1/2  "LateralAcceleration"
  Bus Assignment1/1 -> MotionBaseInputAdapter/2(DynamicsInput)
  Min/1 -> Product2/1
  Constant/1 -> Min/1
  OR/1 -> Data Type Conversion7/1
  Ground/1 -> SR Latch - Set Priority/2
  SR Latch - Set Priority/1 -> Gain5/1
  Gain5/1 -> Product2/3
  BogieDerailedEndImage/1 -> OR/1
  Dynamics In/1 -> Terminator/1
  OnRoughTrackFix/1 -> Bus Assignment/2
  Constant1/1 -> Add1/2

== system BEML_EMU/InputsInterface/FaultHandler/Subsystem/DoorFaults ==
  In Bus Element2 : Inport  PortName=VehicleFaults  Element=TrainDoorNotClosingAtPlatform
  In Bus Element4 : Inport  PortName=VehicleFaults  Element=DoorMajorFault
  In Bus Element5 : Inport  PortName=VehicleFaults  Element=DoorDCUFailure
  In Bus Element6 : Inport  PortName=VehicleFaults  Element=DoorMotorCircuitFailure
  In Bus Element8 : Inport  PortName=VehicleFaults  Element=DoorUnexpectedUnlocking
  In Bus Element9 : Inport  PortName=VehicleFaults  Element=DoorFailedToLock
  In Bus Element10 : Inport  PortName=VehicleFaults  Element=DoorFailedToUnlock
  In Bus Element11 : Inport  PortName=VehicleFaults  Element=DCSRFailure
  In Bus Element12 : Inport  PortName=VehicleFaults  Element=DLSLFailure
  In Bus Element13 : Inport  PortName=VehicleFaults  Element=DLSRFailure
  In Bus Element15 : Inport  PortName=VehicleFaults  Element=UnexpectedDoorOpeningDetectedByCC
  In Bus Element14 : Inport  PortName=VehicleFaults  Element=DCSLFailure
  In Bus Element7 : Inport  PortName=VehicleFaults  Element=EmergencyDoorMechanicalUnlocked
  In Bus Element16 : Inport  PortName=VehicleFaults  Element=DM1A1DoorNotOpeningAtPlatform
  In Bus Element3 : Inport  PortName=VehicleFaults  Element=DoorEmergencyHandleActivation
  In Bus Element : Inport  PortName=VehicleFaults  Element=DoorCloseObstruction
  In Bus Element1 : Inport  PortName=VehicleFaults  Element=DoorOpenObstruction
  Bus Assignment : BusAssignment  AssignedSignals=ObjectObstructingDoorWhileClosing,ObjectObstructingDoorWhileOpening,DoorFailToClose,DoorFailToOpen,DoorMotorCircuitFailure,DoorFailedToLock,DoorFailedToUnlock,DoorUnexpectedUnlocking,DoorDCUFailure,DCSRFailure,DCSLFailure,DLSRFailure,DLSLFailure,DoorMajorFault,UnexpectedDoorOpeningDetectedByCC,EmergencyDoorMechanicalUnlocked,DoorEmergencyHandleActivation
  Constant1 : Constant  Value=0  OutDataTypeStr=Bus: BD_DoorSystem_In_Door_Faults
  Out1 : Outport
  wires:
  Constant1/1 -> Bus Assignment/1
  Bus Assignment/1 -> Out1/1
  In Bus Element/1 -> Bus Assignment/2
  In Bus Element1/1 -> Bus Assignment/3
  In Bus Element2/1 -> Bus Assignment/4
  In Bus Element16/1 -> Bus Assignment/5
  In Bus Element6/1 -> Bus Assignment/6
  In Bus Element9/1 -> Bus Assignment/7
  In Bus Element10/1 -> Bus Assignment/8
  In Bus Element8/1 -> Bus Assignment/9
  In Bus Element5/1 -> Bus Assignment/10
  In Bus Element11/1 -> Bus Assignment/11
  In Bus Element14/1 -> Bus Assignment/12
  In Bus Element13/1 -> Bus Assignment/13
  In Bus Element12/1 -> Bus Assignment/14
  In Bus Element4/1 -> Bus Assignment/15
  In Bus Element15/1 -> Bus Assignment/16
  In Bus Element7/1 -> Bus Assignment/17
  In Bus Element3/1 -> Bus Assignment/18
